simulink model "chap9_3sim"  (Simulink 5.0)
settings: Solver=ode1  StartTime=0.0  StopTime=10  FixedStep=0.001  RelTol=1e-3
libraries: simulink x1
settings Model: LastModifiedBy=Administrator  ExtModeTrigMode=oneshot  ExtModeArmWhenConnect=off  LimitDataPoints=off  BooleanDataType=off

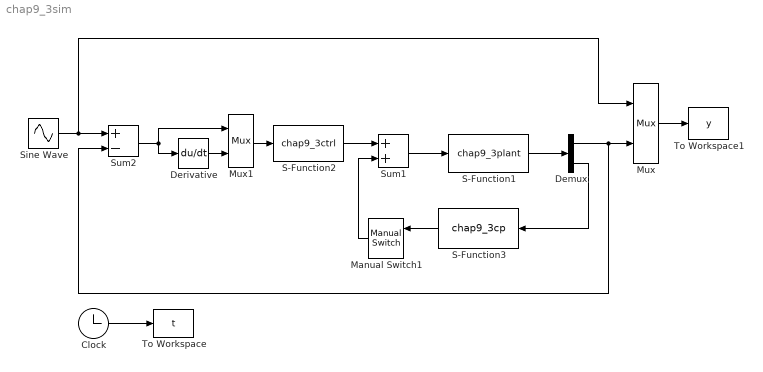
== system chap9_3sim ==
  Clock : Clock
      settings: Decimation=10
  Demux : Demux  Outputs=2
  Derivative : Derivative
  Manual Switch1 : simulink/Signal Routing/Manual Switch  Orientation=left  sw=0  action=0
  Mux : Mux  Inputs=2
  Mux1 : Mux  Inputs=2
  S-Function1 : S-Function  FunctionName=chap9_3plant
  S-Function2 : S-Function  FunctionName=chap9_3ctrl
  S-Function3 : S-Function  Orientation=left  FunctionName=chap9_3cp
  Sine Wave : Sin  Amplitude=0.1  SampleTime=0
  Sum1 : Sum  SaturateOnIntegerOverflow=on  InputSameDT=on
  Sum2 : Sum  Inputs=+-  SaturateOnIntegerOverflow=on  InputSameDT=on
  To Workspace : ToWorkspace  VariableName=t  SampleTime=-1  SaveFormat=Array
  To Workspace1 : ToWorkspace  VariableName=y  SampleTime=-1  SaveFormat=Array
  wires:
  Mux/1 -> To Workspace1/1
  Sine Wave/1 -> Sum2/1, Mux/1
  Clock/1 -> To Workspace/1
  Sum2/1 -> Mux1/1, Derivative/1
  Mux1/1 -> S-Function2/1
  Derivative/1 -> Mux1/2
  S-Function1/1 -> Demux/1
  Demux/1 -> Mux/2, Sum2/2
  Demux/2 -> S-Function3/1
  S-Function3/1 -> Manual Switch1/1
  S-Function2/1 -> Sum1/1
  Manual Switch1/1 -> Sum1/2
  Sum1/1 -> S-Function1/1
